simulink model "Radiator_LM2596"  (R2015b)
settings: Solver=VariableStepAuto  StartTime=0.0  StopTime=100.0  RelTol=1e-3
libraries: fl_lib x15, nesl_utility x5, elec_lib x2
settings Model: Creator=dominikguz  LastModifiedBy=dominikguz
settings DataIOCC: InspectSignalLogs=on

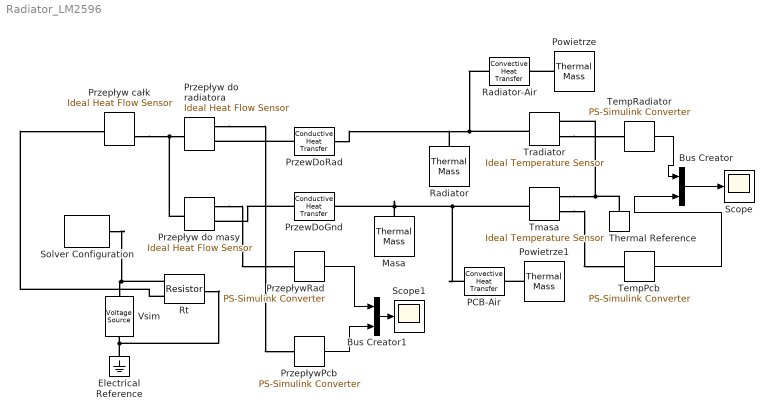
== system Radiator_LM2596 ==
  Bus Creator : BusCreator  Inputs=2
  Bus Creator1 : BusCreator  Inputs=2
  Electrical Reference : fl_lib/Electrical/Electrical Elements/Electrical Reference
  Masa : fl_lib/Thermal/Thermal Elements/Thermal Mass  Description=GND plane  mass=10 g  sp_heat=24 J/kg/K  Q_specify=off  Q_priority=None  Q=0 J/s  T_specify=off  T_priority=None  T=300 K
  "PCB-Air " : fl_lib/Thermal/Thermal Elements/Convective Heat Transfer  area=18 cm^2  heat_tr_coeff=10.45 W/(m^2 * K)  Q_specify=off  Q_priority=None  Q=0 J/s  T_specify=off  T_priority=None  T=0 K
  Powietrze : fl_lib/Thermal/Thermal Elements/Thermal Mass  mass=1.4960e+03 kg  sp_heat=1.0054e+03 J/kg/K  Q_specify=off  Q_priority=None  Q=0 J/s  T_specify=off  T_priority=None  T=300 K
  Powietrze1 : fl_lib/Thermal/Thermal Elements/Thermal Mass  mass=1.4960e+03 kg  sp_heat=1.0054e+03 J/kg/K  Q_specify=off  Q_priority=None  Q=0 J/s  T_specify=off  T_priority=None  T=300 K
  Przepływ całk : fl_lib/Thermal/Thermal Sensors/Ideal Heat Flow Sensor
  Przepływ do masy : fl_lib/Thermal/Thermal Sensors/Ideal Heat Flow Sensor
  Przepływ do radiatora : fl_lib/Thermal/Thermal Sensors/Ideal Heat Flow Sensor
  PrzepływPcb : nesl_utility/PS-Simulink Converter  PhysicalDomain=network_engine_domain  SubClassName=ps_output  LeftPortType=input  RightPortType=output  PseudoPeriodic=off  Frequencies=[]  Unit=1  AffineConversion=on
  PrzepływRad : nesl_utility/PS-Simulink Converter  PhysicalDomain=network_engine_domain  SubClassName=ps_output  LeftPortType=input  RightPortType=output  PseudoPeriodic=off  Frequencies=[]  Unit=1  AffineConversion=on
  PrzewDoGnd : fl_lib/Thermal/Thermal Elements/Conductive Heat Transfer  area=2 mm^2  thickness=5 mm  th_cond=1 W/(m*K)  Q_specify=off  Q_priority=None  Q=0 J/s  T_specify=off  T_priority=None  T=0 K
  PrzewDoRad : fl_lib/Thermal/Thermal Elements/Conductive Heat Transfer  area=2 cm^2  thickness=0.5 mm  th_cond=1 W/(m*K)  Q_specify=off  Q_priority=None  Q=0 J/s  T_specify=off  T_priority=None  T=0 K
  "Radiator " : fl_lib/Thermal/Thermal Elements/Thermal Mass  mass=10 g  sp_heat=24 J/kg/K  Q_specify=off  Q_priority=None  Q=0 J/s  T_specify=off  T_priority=None  T=300 K
  "Radiator-Air " : fl_lib/Thermal/Thermal Elements/Convective Heat Transfer  area=20 cm^2  heat_tr_coeff=52 W/(m^2 * K)  Q_specify=off  Q_priority=None  Q=0 J/s  T_specify=off  T_priority=None  T=0 K
  "Rt " : elec_lib/Passive Devices/Resistor  R=1 Ohm  R_tol=1  enable_R_tol=0  tol_distribution=1  nSigma=4  enable_operating_limits=0  operating_limit_action=2  power_rating=1 W  max_working_voltage=100 V  enable_faults=0  fault_action=1  R_faulted=Inf Ohm  enable_temporal_fault=0  t_fault=1 s  enable_behavioral_fault=0  max_permissible_current=1 A  t_fail_on_current=1 s  noise_mode=0  sample_time=0.001 s  repeatability=1  auto_seed=2843309574  user_seed=0  Tdevice=25 C  alpha=0.00393 1/K  Tmeas=25 C  thermal_mass=2 J/K  initial_temperature=25 C  power_derating_T1=70 C  power_derating_T2=155 C  operating_temperature_range_vec=[ -50 150 ] C
  Scope : Scope
  Scope1 : Scope
  Solver Configuration : nesl_utility/Solver Configuration  PhysicalDomain=network_engine_domain  SubClassName=solver  LeftPortType=input  RightPortType=generic  Accelerate=off  Tones=[]  Harmonics=[]  SimulateNoise=off  Profile=off  UseLocalSampling=off  EnableSwitchedLinearOptims=on  FrequencyDomain=off  UseCCode=off  RelTol=0.001  AbsTol=1e-06  MinStep=1e-09  ToWorkspace=off  RevertToSquareIcSolve=off  NumHomotopyIterations=100  PhasorMode=off  PhasorModeNumHarmonics=1  DoDC=off  ResidualTolerance=1e-09  UseLocalSolver=off  LocalSolverChoice=NE_BACKWARD_EULER_ADVANCER  LocalSolverSampleTime=0.001  DoFixedCost=off  MaxNonlinIter=3  MaxModeIter=2  LinearAlgebra=Sparse  DelaysMemoryBudget=1024  AutomaticFiltering=on  FilteringTimeConstant=0.001
  TempPcb : nesl_utility/PS-Simulink Converter  PhysicalDomain=network_engine_domain  SubClassName=ps_output  LeftPortType=input  RightPortType=output  PseudoPeriodic=off  Frequencies=[]  Unit=C  AffineConversion=on
  TempRadiator : nesl_utility/PS-Simulink Converter  PhysicalDomain=network_engine_domain  SubClassName=ps_output  LeftPortType=input  RightPortType=output  PseudoPeriodic=off  Frequencies=[]  Unit=C  AffineConversion=on
  Thermal Reference : fl_lib/Thermal/Thermal Elements/Thermal Reference
  Tmasa : fl_lib/Thermal/Thermal Sensors/Ideal Temperature Sensor
  Tradiator : fl_lib/Thermal/Thermal Sensors/Ideal Temperature Sensor
  "Vsim " : elec_lib/Sources/Voltage Source  dc_voltage=3.18 V  ac_voltage=0 V  ac_shift=0 deg  ac_frequency=60 Hz  noise_mode=0  PSD=0 V^2/Hz  sample_time=0.001 s  repeatability=1  auto_seed=3775335973  user_seed=0
  wires:
  TempRadiator/1 -> Bus Creator/1
  TempPcb/1 -> Bus Creator/2
  Bus Creator/1 -> Scope/1
  PrzepływRad/1 -> Bus Creator1/1
  PrzepływPcb/1 -> Bus Creator1/2
  Bus Creator1/1 -> Scope1/1
  connections:
  Tradiator/LConn1 -- PrzewDoRad/RConn1 -- "Radiator "/LConn1 -- "Radiator-Air "/LConn1
  Tmasa/LConn1 -- "PCB-Air "/LConn1 -- Masa/LConn1 -- PrzewDoGnd/RConn1
  Przepływ do masy/LConn1 -- Przepływ całk/RConn2 -- Przepływ do radiatora/LConn1
  PrzewDoGnd/LConn1 -- Przepływ do masy/RConn2
  Tmasa/RConn1 -- Thermal Reference/LConn1 -- Tradiator/RConn1
  "Rt "/LConn1 -- Solver Configuration/RConn1 -- "Vsim "/LConn1
  "Rt "/RConn1 -- Electrical Reference/LConn1 -- "Vsim "/RConn1
  Powietrze/LConn1 -- "Radiator-Air "/RConn1
  Tradiator/RConn2 -- TempRadiator/LConn1
  Tmasa/RConn2 -- TempPcb/LConn1
  "Rt "/LConn2 -- Przepływ całk/LConn1
  Powietrze1/LConn1 -- "PCB-Air "/RConn1
  Przepływ do radiatora/RConn1 -- PrzepływPcb/LConn1
  PrzewDoRad/LConn1 -- Przepływ do radiatora/RConn2
  Przepływ do masy/RConn1 -- PrzepływRad/LConn1
